simulink model "dspconstant_tut"  (Simulink 4.00)
settings: Solver=FixedStepDiscrete  StartTime=0.0  StopTime=10.0  RelTol=1e-3
PostLoadFcn:
  | set_param(gcs,'SimulationCommand','Update')
libraries: dspsrcs3 x5
settings Model: RequirementInfo=9  LastModifiedBy=dfass  LimitDataPoints=off  ExtModeTrigMode=oneshot  ExtModeArmWhenConnect=off  BlockReductionOpt=off

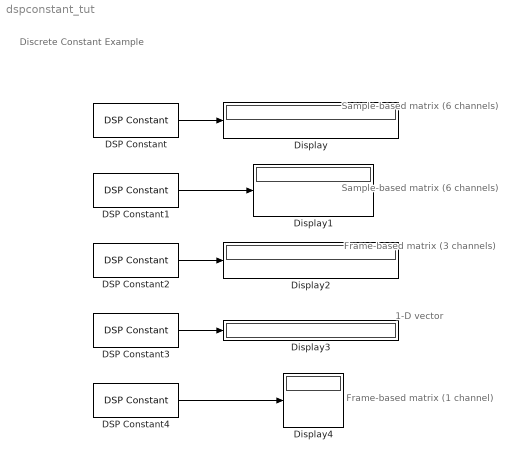
== system dspconstant_tut ==
  note: Discrete Constant Example
  note: Sample-based matrix
      | (6 channels)
  note: Sample-based matrix
      | (6 channels)
  note: Frame-based matrix
      | (3 channels)
  note: 1-D vector
  note: Frame-based matrix
      | (1 channel)
  DSP Constant : dspsrcs3/DSP Constant  Value=[1 2 3;4 5 6]  InterpretAs1D=off  SampleMode=Discrete  Ts=1  FramebasedOutput=off
  DSP Constant1 : dspsrcs3/DSP Constant  Value=[1 2 3;4 5 6]'  InterpretAs1D=off  SampleMode=Discrete  Ts=1  FramebasedOutput=off
  DSP Constant2 : dspsrcs3/DSP Constant  Value=randn(2,3)  InterpretAs1D=off  SampleMode=Discrete  Ts=1  FramebasedOutput=on
  DSP Constant3 : dspsrcs3/DSP Constant  Value=[1 2 3]  InterpretAs1D=on  SampleMode=Discrete  Ts=1  FramebasedOutput=off
  DSP Constant4 : dspsrcs3/DSP Constant  Value=[1 2 3]'  InterpretAs1D=off  SampleMode=Discrete  Ts=1  FramebasedOutput=on
  Display{,1..4} (5 alike) : Display
      settings: Format=short
  wires:
  DSP Constant/1 -> Display/1
  DSP Constant1/1 -> Display1/1
  DSP Constant2/1 -> Display2/1
  DSP Constant3/1 -> Display3/1
  DSP Constant4/1 -> Display4/1
